simulink model "ts"  (R2020b)
settings: Solver=ode4  StartTime=0.0  StopTime=5  FixedStep=1/400  RelTol=1e-3
libraries: discretizing x3
settings Model: Creator=kcx06  LastModifiedBy=kcx06

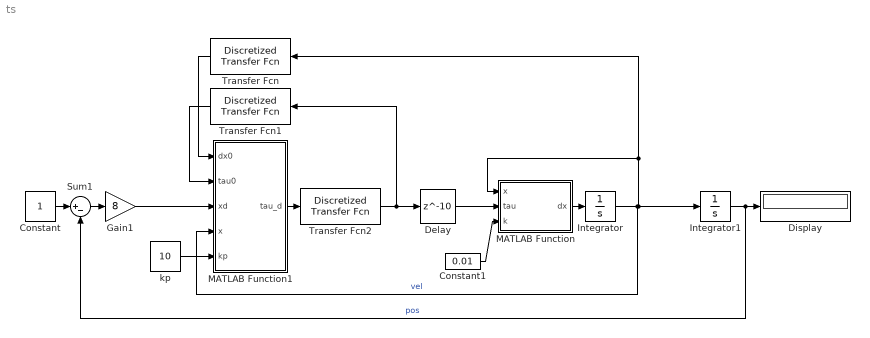
== system ts ==
  Constant : Constant
  Constant1 : Constant  Value=0.01
  Delay : Delay  DelayLength=10
  Display : Display
  Gain1 : Gain  Gain=8
  Integrator : Integrator
  Integrator1 : Integrator
  MATLAB Function : MATLAB Function  TreatAsAtomicUnit=on
  MATLAB Function1 : MATLAB Function  TreatAsAtomicUnit=on
  Sum1 : Sum  Inputs=|+-
  Transfer Fcn : discretizing/Discretized Transfer Fcn  Numerator=[1 0]  Denominator=[0.06 1]  AbsTol=auto  SampleTime=1/400  method=zoh  Wc=1
      settings: SourceProductBaseCode=SL
  Transfer Fcn1 : discretizing/Discretized Transfer Fcn  Numerator=[1]  Denominator=[0.06 1]  AbsTol=auto  SampleTime=1/400  method=zoh  Wc=1
      settings: SourceProductBaseCode=SL
  Transfer Fcn2 : discretizing/Discretized Transfer Fcn  Numerator=[1]  Denominator=[0.035 1]  AbsTol=auto  SampleTime=1/400  method=zoh  Wc=1
      settings: SourceProductBaseCode=SL
  kp : Constant  Value=10
  wires:
  Sum1/1 -> Gain1/1
  MATLAB Function/1(dx) -> Integrator/1
  Integrator/1 -> Transfer Fcn/1, MATLAB Function/1(x), Integrator1/1, MATLAB Function1/4(x)  "vel"
  Constant1/1 -> MATLAB Function/3(k)
  Integrator1/1 -> Sum1/2, Display/1  "pos"
  Constant/1 -> Sum1/1
  MATLAB Function1/1(tau_d) -> Transfer Fcn2/1
  Transfer Fcn/1 -> MATLAB Function1/1(dx0)
  Transfer Fcn1/1 -> MATLAB Function1/2(tau0)
  kp/1 -> MATLAB Function1/5(kp)
  Gain1/1 -> MATLAB Function1/3(xd)
  Transfer Fcn2/1 -> Delay/1, Transfer Fcn1/1
  Delay/1 -> MATLAB Function/2(tau)

== matlab function ts/MATLAB Function1 ==
  data: dx0 input; tau_d output; tau0 input; xd input; x input; kp input
function tau_d = fcn(dx0, tau0, xd, x, kp)
tau_d = tau0 + kp*(xd-x) - dx0;

== matlab function ts/MATLAB Function ==
  data: x input; dx output; tau input; k input
function dx = fcn(x, tau,k)
dx = -k*x + tau;
